simulink model "Simulation_P2_r2023a"  (R2023a)
settings: Solver=FixedStepAuto  StartTime=0.0  StopTime=10  FixedStep=1e-3  RelTol=1e-3  EnableMultiTasking=on
undefined symbols (not defined in the file): A0, A1, D0, D1, D10, D11, D12, D13, D2, D3, D4, D5, D6, D7, D8, D9, magnitude, PTA0, PTA1, PTA2, PTB2, PTB23, PTB3, PTB9, PTC16, PTC17, PTC2, PTC3, PTC4, PTD0, PTD1, PTD2, PTD3
libraries: frdmk64flib x20, etargetslib x18, dspstat3 x1
settings Model: ExtModeTrigDuration=5  Creator=sherr  LastModifiedBy=salihahussain
settings OptimizationCC: EnhancedBackFolding=on  PassReuseOutputArgsAs=Individual arguments  ZeroExternalMemoryAtStartup=off  ZeroInternalMemoryAtStartup=off  MaxStackSize=64  OptimizeBlockOrder=speed  DifferentSizesBufferReuse=on  OptimizationCustomize=off  EfficientTunableParamExpr=on
settings DebuggingCC: ParameterTunabilityLossMsg=error
settings HardwareCC: ProdBitPerPointer=32  ProdBitPerSizeT=32  ProdBitPerPtrDiffT=32  ProdLargestAtomicInteger=Long  ProdLargestAtomicFloat=Double  ProdWordSize=32  ProdHWDeviceType=ARM Compatible->ARM Cortex
settings SFSimCC: MATLABDynamicMemAlloc=off
settings RTWCC: Description=Embedded Coder  SystemTargetFile=ert.tlc  HardwareBoard=NXP FRDM-K64F  TLCOptions="-aInlineSetEventsForThisBaseRateFcn=TLC_FALSE -aSuppressMultiTaskScheduler=TLC_FALSE  -aRateBasedStepFcn=0"  TemplateMakefile=ert_default_tmf  Toolchain=GNU Tools for ARM Embedded Processors
settings CodeAppCC: ForceParamTrailComments=on  IgnoreCustomStorageClasses=off  OperatorAnnotations=on  SimulinkDataObjDesc=on  SFDataObjDesc=on  InsertBlockDesc=on
settings ERTTargetCC: ExtModeTransport=4  ExtModeMexFile=sendToCommService

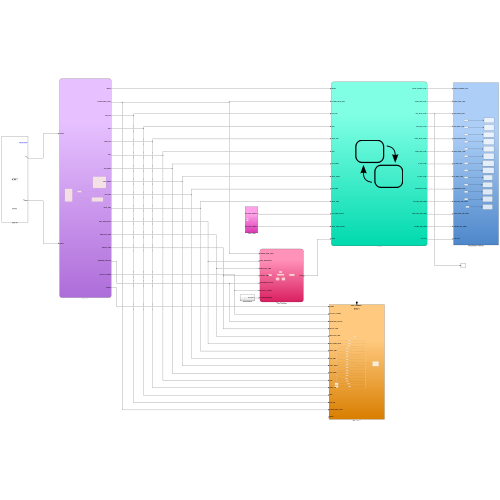
[thumbnail: Simulink's stored preview of the top-level diagram]
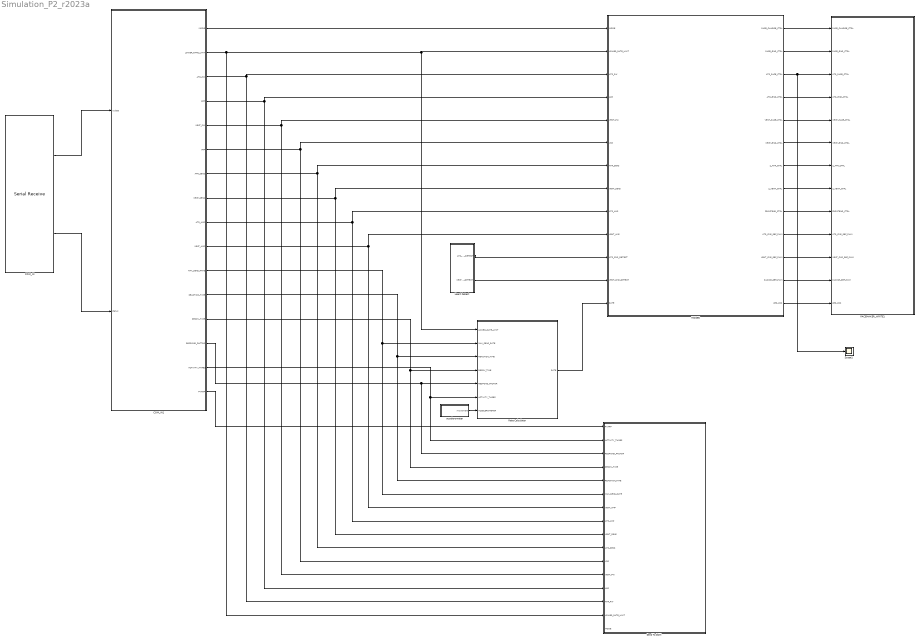
== system Simulation_P2_r2023a ==
  COM_IN : frdmk64flib/Serial Receive  SCIModule=0  Baudrate=uint32(9600)  Parity=None  StopBits=1  HardwareFlowControl=None  ByteOrder=LittleEndian  DataType=uint8  DataLength=10  BlockingMode=off  OutputStatus=on  SampleTime=0.1
  COM_IN1 : Stateflow chart  TreatAsAtomicUnit=on
      settings: PortSchema="{\"entries\":[{\"content\":{\"sides\":[{\"content\":{\"connectorIds\":[\"In1\",\"In2\"]},\"type\":\"ConnectorPlacement.EquallySpacedRectSide\",\"uuid\":\"bacdf752-87eb-4404-babc-2d3eecd8d2c0\"},{\"content\":{\"connectorIds\":[\"Out12\",\"Out7\",\"Out1\",\"Out2\",\"Out3\",\"Out4\",\"Out5\",\"Out6\",\"Out8\",\"Out9\",\"Out11\",\"Out13\",\"Out14\",\"Out15\",\"Out16\",\"Out10\"],\"side\":\"RIGHT\"},\"type\":\"ConnectorPlacement.EquallySpacedRectSide\",\"uuid\":\"87a5995d-41f9-45bd-b026-59ec7d01c35a\"},{\"content\":{\"side\":\"TOP\"},\"type\":\"ConnectorPlacement.EquallySpacedRectSide\",\"uuid\":\"9c1d1ff9-71c1-4ac7-ac77-ae13538ca481\"}]},\"type\":\"ConnectorPlacement.EquallySpacedConnector\",\"uuid\":\"f58684e7-fbf2-4992-a059-d31a56d65e02\"}],\"packageUris\":[\"http://schema.mathworks.com/mf0/Connector/R2020b\"],\"version\":\"1.0\"}"
  Heart Detect : Subsystem
  MODES : Stateflow chart  TreatAsAtomicUnit=on
  PACEMAKER_WRITE1 : Subsystem
  Rate Calculator : Stateflow chart  TreatAsAtomicUnit=on
      settings: PortSchema="{\"entries\":[{\"content\":{\"sides\":[{\"content\":{\"connectorIds\":[\"In3\",\"In7\",\"In5\",\"In4\",\"In1\",\"In2\",\"In6\"]},\"type\":\"ConnectorPlacement.EquallySpacedRectSide\",\"uuid\":\"c5d5357b-99af-427e-a4c2-6249b97164da\"},{\"content\":{\"connectorIds\":[\"Out1\"],\"side\":\"RIGHT\"},\"type\":\"ConnectorPlacement.EquallySpacedRectSide\",\"uuid\":\"358f3739-9c7f-4556-a3f3-e36ee066d1ea\"},{\"content\":{\"connectorIds\":[],\"side\":\"TOP\"},\"type\":\"ConnectorPlacement.EquallySpacedRectSide\",\"uuid\":\"e7873f65-b91d-40fa-bd89-8dce436ca138\"}]},\"type\":\"ConnectorPlacement.EquallySpacedConnector\",\"uuid\":\"f1b9a7e0-0d96-4ba5-9c87-c58b64bb2144\"}],\"packageUris\":[\"http://schema.mathworks.com/mf0/Connector/R2020b\"],\"version\":\"1.0\"}"
  Scope1 : Scope
  Send To DCM : Subsystem
  accelerometer : Subsystem
  wires:
  COM_IN/2 -> COM_IN1/2(status)
  COM_IN/1 -> COM_IN1/1(rxdata)
  MODES/10(ATR_CMP_REF_PWM) -> PACEMAKER_WRITE1/10(ATR_CMP_REF_PWM)
  MODES/2(PACE_GND_CTRL) -> PACEMAKER_WRITE1/2(PACE_GND_CTRL)
  MODES/6(VENT_GND_CTRL) -> PACEMAKER_WRITE1/6(VENT_GND_CTRL)
  MODES/11(VENT_CMP_REF_PWM) -> PACEMAKER_WRITE1/11(VENT_CMP_REF_PWM)
  MODES/9(FRONTEND_CTRL) -> PACEMAKER_WRITE1/9(FRONTEND_CTRL)
  MODES/13(LED_C22) -> PACEMAKER_WRITE1/13(LED_C22)
  MODES/1(PACE_CHARGE_CTRL) -> PACEMAKER_WRITE1/1(PACE_CHARGE_CTRL)
  MODES/7(Z_ATR_CTRL) -> PACEMAKER_WRITE1/7(Z_ATR_CTRL)
  MODES/4(ATR_GND_CTRL) -> PACEMAKER_WRITE1/4(ATR_GND_CTRL)
  MODES/5(VENT_PACE_CTRL) -> PACEMAKER_WRITE1/5(VENT_PACE_CTRL)
  MODES/12(PACING_REF_PWM) -> PACEMAKER_WRITE1/12(PACING_REF_PWM)
  MODES/8(Z_VENT_CTRL) -> PACEMAKER_WRITE1/8(Z_VENT_CTRL)
  MODES/3(ATR_PACE_CTRL) -> Scope1/1, PACEMAKER_WRITE1/3(ATR_PACE_CTRL)
  COM_IN1/9(VENT_AMP) -> Send To DCM/7(VENT_AMP), MODES/10(VENT_AMP)
  Heart Detect/1(ATR_CMP_DETECT) -> MODES/11(ATR_CMP_DETECT)
  Heart Detect/2(VENT_CMP_DETECT) -> MODES/12(VENT_CMP_DETECT)
  COM_IN1/12(MODE) -> MODES/1(MODE)
  COM_IN1/8(ATR_AMP) -> Send To DCM/8(ATR_AMP), MODES/9(ATR_AMP)
  COM_IN1/6(VENT_SENS) -> Send To DCM/9(VENT_SENS), MODES/8(VENT_SENS)
  COM_IN1/5(ATR_SENS) -> Send To DCM/10(ATR_SENS), MODES/7(ATR_SENS)
  COM_IN1/4(VRP) -> Send To DCM/11(VRP), MODES/6(VRP)
  COM_IN1/3(VENT_PW) -> Send To DCM/12(VENT_PW), MODES/5(VENT_PW)
  COM_IN1/2(ARP) -> Send To DCM/13(ARP), MODES/4(ARP)
  COM_IN1/1(ATR_PW) -> Send To DCM/14(ATR_PW), MODES/3(ATR_PW)
  COM_IN1/7(LOWER_RATE_LIMIT) -> Send To DCM/15(LOWER_RATE_LIMIT), Rate Calculator/3(LOWER_RATE_LIMIT), MODES/2(LOWER_RATE_LIMIT)
  COM_IN1/11(MAX_SENS_RATE) -> Send To DCM/6(MAX_SENS_RATE), Rate Calculator/7(MAX_SENS_RATE)
  COM_IN1/13(REACTION_TIME) -> Send To DCM/5(REACTION_TIME), Rate Calculator/5(REACTION_TIME)
  COM_IN1/14(RECOV_TIME) -> Send To DCM/4(RECOV_TIME), Rate Calculator/4(RECOV_TIME)
  COM_IN1/15(RESPOND_FACTOR) -> Send To DCM/3(RESPOND_FACTOR), Rate Calculator/1(RESPOND_FACTOR)
  COM_IN1/16(ACTIVITY_THRES) -> Send To DCM/2(ACTIVITY_THRES), Rate Calculator/2(ACTIVITY_THRES)
  accelerometer/1(movement) -> Rate Calculator/6(ACCELEROMETER)
  COM_IN1/10(PVARP) -> Send To DCM/1(PVARP)
  Rate Calculator/1(RATE) -> MODES/13(RATE)

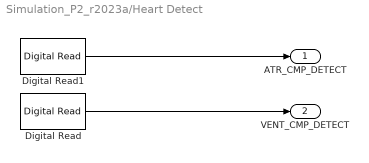
== system Simulation_P2_r2023a/Heart Detect ==
  Digital Read : frdmk64flib/Digital Read  Whichpin=PTC17 (D1)  SampleTime=-1
  Digital Read1 : frdmk64flib/Digital Read  Whichpin=PTC16 (D0)  SampleTime=-1
  ATR_CMP_DETECT : Outport
  VENT_CMP_DETECT : Outport  Port=2
  wires:
  Digital Read/1 -> VENT_CMP_DETECT/1
  Digital Read1/1 -> ATR_CMP_DETECT/1

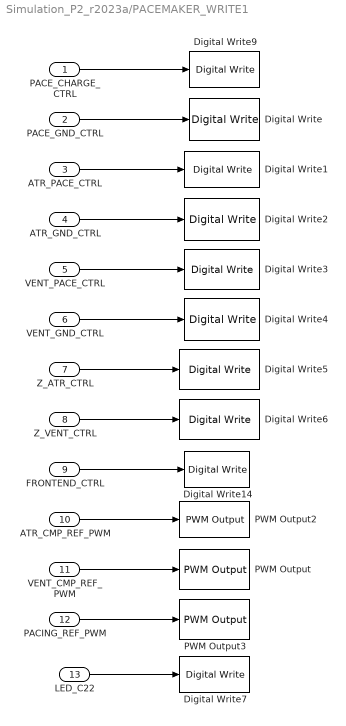
== system Simulation_P2_r2023a/PACEMAKER_WRITE1 ==
  PACE_CHARGE_CTRL : Inport
  PACE_GND_CTRL : Inport  Port=2
  ATR_PACE_CTRL : Inport  Port=3
  ATR_GND_CTRL : Inport  Port=4
  VENT_PACE_CTRL : Inport  Port=5
  VENT_GND_CTRL : Inport  Port=6
  Z_ATR_CTRL : Inport  Port=7
  Z_VENT_CTRL : Inport  Port=8
  FRONTEND_CTRL : Inport  Port=9
  ATR_CMP_REF_PWM : Inport  Port=10
  VENT_CMP_REF_PWM : Inport  Port=11
  PACING_REF_PWM : Inport  Port=12
  LED_C22 : Inport  Port=13
  Digital Write : frdmk64flib/Digital Write  Whichpin=PTD0 (D10)
  Digital Write1 : frdmk64flib/Digital Write  Whichpin=PTA0 (D8)
  Digital Write14 : frdmk64flib/Digital Write  Whichpin=PTD1 (D13)
  Digital Write2 : frdmk64flib/Digital Write  Whichpin=PTD2 (D11)
  Digital Write3 : frdmk64flib/Digital Write  Whichpin=PTC4 (D9)
  Digital Write4 : frdmk64flib/Digital Write  Whichpin=PTD3 (D12)
  Digital Write5 : frdmk64flib/Digital Write  Whichpin=PTB23 (D4)
  Digital Write6 : frdmk64flib/Digital Write  Whichpin=PTC3 (D7)
  Digital Write7 : frdmk64flib/Digital Write  Whichpin=BLUE_LED
  Digital Write9 : frdmk64flib/Digital Write  Whichpin=PTB9 (D2)
  PWM Output : frdmk64flib/PWM Output  Whichpin=PTA1 (D3)  InitialFrequency=2000  InitialDutyCycle=100
  PWM Output2 : frdmk64flib/PWM Output  Whichpin=PTC2 (D6)  InitialFrequency=2000  InitialDutyCycle=100
  PWM Output3 : frdmk64flib/PWM Output  Whichpin=PTA2 (D5)  InitialFrequency=2000  InitialDutyCycle=100
  wires:
  PACE_GND_CTRL/1 -> Digital Write/1
  ATR_CMP_REF_PWM/1 -> PWM Output2/1
  Z_ATR_CTRL/1 -> Digital Write5/1
  ATR_GND_CTRL/1 -> Digital Write2/1
  Z_VENT_CTRL/1 -> Digital Write6/1
  FRONTEND_CTRL/1 -> Digital Write14/1
  PACE_CHARGE_CTRL/1 -> Digital Write9/1
  VENT_GND_CTRL/1 -> Digital Write4/1
  PACING_REF_PWM/1 -> PWM Output3/1
  ATR_PACE_CTRL/1 -> Digital Write1/1
  VENT_CMP_REF_PWM/1 -> PWM Output/1
  VENT_PACE_CTRL/1 -> Digital Write3/1
  LED_C22/1 -> Digital Write7/1

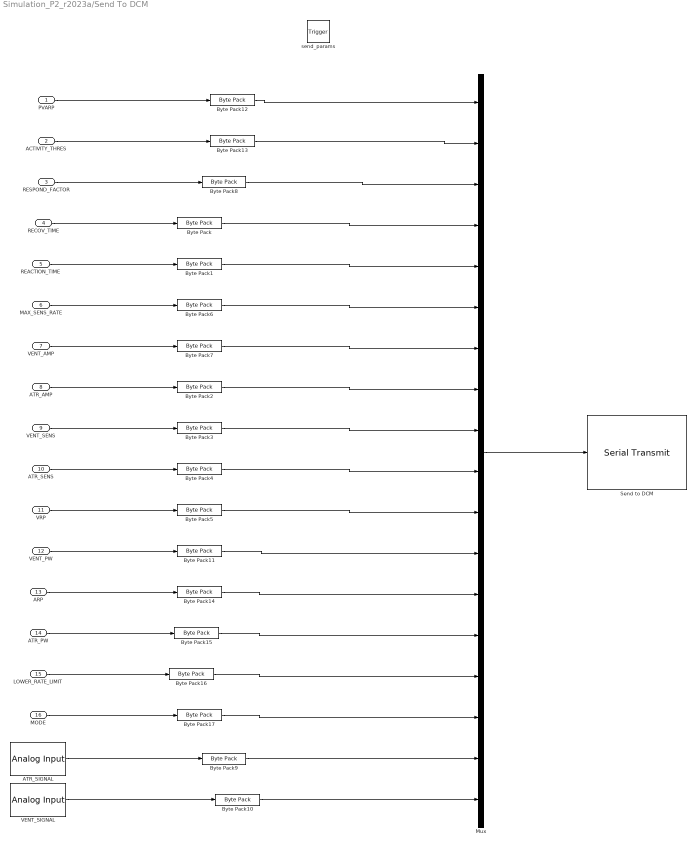
== system Simulation_P2_r2023a/Send To DCM ==
  PVARP : Inport
  ACTIVITY_THRES : Inport  Port=2
  RESPOND_FACTOR : Inport  Port=3
  RECOV_TIME : Inport  Port=4
  REACTION_TIME : Inport  Port=5
  MAX_SENS_RATE : Inport  Port=6
  VENT_AMP : Inport  Port=7
  ATR_AMP : Inport  Port=8
  VENT_SENS : Inport  Port=9
  ATR_SENS : Inport  Port=10
  VRP : Inport  Port=11
  VENT_PW : Inport  Port=12
  ARP : Inport  Port=13
  ATR_PW : Inport  Port=14
  LOWER_RATE_LIMIT : Inport  Port=15
  MODE : Inport  Port=16
  send_params : TriggerPort  TriggerType=function-call  IsSimulinkFunction=on  FunctionName=send_params  VariantControl=(inherit)  PortDimensions=1
  ATR_SIGNAL : frdmk64flib/Analog Input  Whichpin=PTB2 (A0)  SampleTime=-1
  Byte Pack{,1..3,6..7} (6 alike) : etargetslib/Byte Pack  datatypes={'single'}  byteAlign=1
  Byte Pack10 : etargetslib/Byte Pack  datatypes={'double'}  byteAlign=1
  Byte Pack{4..5,8,11..17} (10 alike) : etargetslib/Byte Pack  datatypes={'uint16'}  byteAlign=1
  Byte Pack9 : etargetslib/Byte Pack  datatypes={'double'}  byteAlign=1
  Mux : Mux  Inputs=18
  Send to DCM : frdmk64flib/Serial Transmit  SCIModule=0  Baudrate=uint32(9600)  Parity=None  StopBits=1  HardwareFlowControl=None  ByteOrder=LittleEndian  BlockingMode=on  OutputStatus=off
  VENT_SIGNAL : frdmk64flib/Analog Input  Whichpin=PTB3 (A1)  SampleTime=-1
  wires:
  PVARP/1 -> Byte Pack12/1
  ACTIVITY_THRES/1 -> Byte Pack13/1
  RECOV_TIME/1 -> Byte Pack/1
  Byte Pack/1 -> Mux/4
  REACTION_TIME/1 -> Byte Pack1/1
  Byte Pack1/1 -> Mux/5
  MAX_SENS_RATE/1 -> Byte Pack6/1
  VENT_AMP/1 -> Byte Pack7/1
  ATR_AMP/1 -> Byte Pack2/1
  Byte Pack2/1 -> Mux/8
  VENT_SENS/1 -> Byte Pack3/1
  Byte Pack3/1 -> Mux/9
  Byte Pack4/1 -> Mux/10
  ATR_SENS/1 -> Byte Pack4/1
  VRP/1 -> Byte Pack5/1
  Byte Pack5/1 -> Mux/11
  VENT_PW/1 -> Byte Pack11/1
  ARP/1 -> Byte Pack14/1
  ATR_PW/1 -> Byte Pack15/1
  LOWER_RATE_LIMIT/1 -> Byte Pack16/1
  MODE/1 -> Byte Pack17/1
  Mux/1 -> Send to DCM/1
  Byte Pack6/1 -> Mux/6
  Byte Pack7/1 -> Mux/7
  RESPOND_FACTOR/1 -> Byte Pack8/1
  ATR_SIGNAL/1 -> Byte Pack9/1
  VENT_SIGNAL/1 -> Byte Pack10/1
  Byte Pack10/1 -> Mux/18
  Byte Pack8/1 -> Mux/3
  Byte Pack9/1 -> Mux/17
  Byte Pack12/1 -> Mux/1
  Byte Pack13/1 -> Mux/2
  Byte Pack11/1 -> Mux/12
  Byte Pack14/1 -> Mux/13
  Byte Pack15/1 -> Mux/14
  Byte Pack16/1 -> Mux/15
  Byte Pack17/1 -> Mux/16

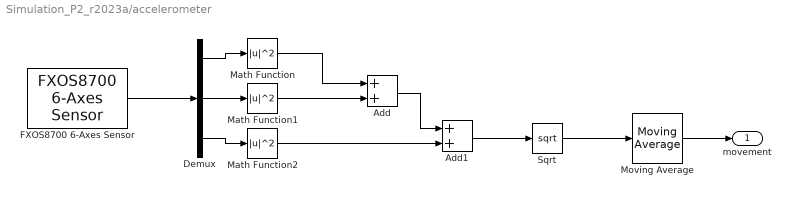
== system Simulation_P2_r2023a/accelerometer ==
  Add : Sum
  Add1 : Sum
  Demux : Demux  Outputs=3
  FXOS8700 6-Axes Sensor : frdmk64flib/FXOS8700 6-Axes Sensor  Activesensor=Accelerometer only  ODR=800Hz  HybridODR=400Hz  Accelfullrange=-4g to +4g  SampleTime=0.01
  Math Function : Math  Operator=magnitude^2
  Math Function1 : Math  Operator=magnitude^2
  Math Function2 : Math  Operator=magnitude^2
  Moving Average : dspstat3/Moving Average  Method=Sliding window  ForgettingFactorPort=off  SpecifyWindowLength=on  WindowLength=500  OverlapLength=499  AllowArbitraryInputLength=off  ForgettingFactor=0.9  SimulateUsing=Code generation
  Sqrt : Sqrt
  movement : Outport
  wires:
  Math Function/1 -> Add/1
  Math Function1/1 -> Add/2
  Math Function2/1 -> Add1/2
  Add/1 -> Add1/1
  Add1/1 -> Sqrt/1
  Sqrt/1 -> Moving Average/1
  Moving Average/1 -> movement/1
  FXOS8700 6-Axes Sensor/1 -> Demux/1
  Demux/1 -> Math Function/1
  Demux/2 -> Math Function1/1
  Demux/3 -> Math Function2/1

== stateflow chart Simulation_P2_r2023a/COM_IN1 ==
  note: Define datatype and size of each variables
  state SET_PARAM
    entry:
    MODE = typecast(rxdata(3:4),'uint16');
    LOWER_RATE_LIMIT = typecast(rxdata(5:6),'uint16');
    ATR_AMP = typecast(rxdata(7:10), 'single');
    ATR_PW = typecast(rxdata(11:14), 'single');
    VENT_AMP = typecast(rxdata(15:18), 'single');
    VENT_PW = typecast(rxdata(19:22), 'single');
    VRP = typecast(rxdata(23:24), 'uint16');
    ARP = typecast(rxdata(25:26), 'uint16');
    MAX_SENS_RATE = typecast(rxdata(27:28), 'uint16');
    ATR_SENS =typecast(rxdata(29:32), 'single');
    VENT_SENS = typecast(rxdata(33:36) ,'single');
    PVARP = typecast(rxdata(37:38), 'uint16');
    ACTIVITY_THRES = typecast(rxdata(39:40), 'uint16');
    REACTION_TIME = typecast(rxdata(41:42), 'uint16');
    RESPOND_FACTOR =typecast(rxdata(43:44), 'uint16');
    RECOV_TIME = typecast(rxdata(45:46), 'uint16');
  note: Set default values
  state INITIAL
    entry:
    MODE = 1; %select any mode
    LOWER_RATE_LIMIT = 60; %ppm
    ATR_AMP = 3.75;
    ATR_PW = 0.4;
    VENT_AMP = 3.75;
    VENT_PW = 0.4;
    VRP = 320;
    ARP = 250;
    MAX_SENS_RATE = 120;
    ATR_SENS = 0.075;%3.75
    VENT_SENS = 0.25;%3.75
    PVARP = 250;
    ACTIVITY_THRES = 0;
    REACTION_TIME = 30;
    RESPOND_FACTOR = 8;
    RECOV_TIME = 2;
  state STANDBY
    %waiting for COM
  state ECHO_PARAM
    entry:
    send_params();
  SET_PARAM -> STANDBY
  (default) -> INITIAL
  (junction 14) -> SET_PARAM [order 1] : [rxdata(2) == hex2dec('55')]
  INITIAL -> STANDBY
  STANDBY -> (junction 15) : [status == 0]
  (junction 15) -> (junction 14) : [rxdata(1) == hex2dec('16')]
  (junction 14) -> ECHO_PARAM [order 2] : [rxdata(2) == hex2dec('22')]
  ECHO_PARAM -> STANDBY
  data: rxdata input uint8; status input uint8; ATR_PW output uint16; ARP output uint16; VENT_PW output single; VRP output single; ATR_SENS output single; VENT_SENS output single; LOWER_RATE_LIMIT output uint16; ATR_AMP output single; VENT_AMP output single; PVARP output uint16; MAX_SENS_RATE output; MODE output uint16; REACTION_TIME output uint16; RECOV_TIME output uint16; RESPOND_FACTOR output uint16; ACTIVITY_THRES output uint16

== stateflow chart Simulation_P2_r2023a/MODES ==
  state INITIAL
    %Initial State
  state AOO [group]
    state CHARGING
      entry:
      %Begin Charging C22 Capacitor
      ATR_PACE_CTRL = 0
      VENT_PACE_CTRL = 0
      PACING_REF_PWM = 100*ATR_AMP/5
      PACE_CHARGE_CTRL = 1
      %Begin Discharging C21 Blocking Capacitor
      PACE_GND_CTRL = 1
      VENT_PACE_CTRL = 0
      Z_ATR_CTRL = 0
      Z_VENT_CTRL = 0
      ATR_PACE_CTRL = 0
      ATR_GND_CTRL = 1
      VENT_GND_CTRL = 0
      %Test
      LED_C22 = 1
    state DISCHARGING
      entry:
      %Discharge C22 into Atrium (AtrialPacing)
      %Begin Charging C21 Blocking Capacitor
      PACE_CHARGE_CTRL = 0
      PACE_GND_CTRL = 1
      ATR_PACE_CTRL = 1
      ATR_GND_CTRL = 0
      Z_ATR_CTRL = 0
      Z_VENT_CTRL = 0
      VENT_GND_CTRL = 0
      VENT_PACE_CTRL  = 0
    AOO.CHARGING -> AOO.DISCHARGING [order 1] : [after(((60000/LOWER_RATE_LIMIT)-ATR_PW), msec)]
    AOO.DISCHARGING -> AOO.CHARGING : [after(ATR_PW, msec)]
  state AAI [group]
    state PROXY
      entry:
      %Discharge C21 Blocking Capacitor
      PACE_GND_CTRL = true;
      VENT_PACE_CTRL = false;
      Z_ATR_CTRL = false;
      Z_VENT_CTRL = false;
      ATR_PACE_CTRL = false;
      ATR_GND_CTRL = true;
      VENT_GND_CTRL = false;
      %Charge C22
      ATR_PACE_CTRL = false;
      VENT_PACE_CTRL = false;
      PACING_REF_PWM = 100*ATR_AMP/5;
      PACE_CHARGE_CTRL = true;
    state CHARGING
      entry:
      %Sensing Circuitry
      FRONTEND_CTRL = HIGH
      %Assume appropriate PWM threshold
      ATR_CMP_REF_PWM = 100*ATR_AMP/5;
      VENT_CMP_REF_PWM = 0
      %Begin Charging C22 Capacitor
      ATR_PACE_CTRL = false;
      VENT_PACE_CTRL = false;
      PACING_REF_PWM = 100*ATR_AMP/5;
      PACE_CHARGE_CTRL = true;
      %Begin Discharging C21 Blocking Capacitor
      PACE_GND_CTRL = true;
      VENT_PACE_CTRL = false;
      Z_ATR_CTRL = false;
      Z_VENT_CTRL = false;
      ATR_PACE_CTRL = false;
      ATR_GND_CTRL = true;
      VENT_GND_CTRL = false;
    state DISCHARGING
      entry:
      %Discharge C22 into Atrium (Atrial Pacing)
      %Begin Charging Blocking Capacitor
      PACE_CHARGE_CTRL = LOW
      PACE_GND_CTRL = HIGH
      ATR_PACE_CTRL = HIGH
      ATR_GND_CTRL = LOW
      Z_ATR_CTRL = LOW
      Z_VENT_CTRL = LOW
      VENT_GND_CTRL = LOW
      VENT_PACE_CTRL  = LOW
    AAI.DISCHARGING -> AAI.PROXY : [after(ATR_PW, msec)]
    AAI.PROXY -> AAI.CHARGING : [after(ARP, msec)]
    (junction 116) -> AAI.PROXY : [after(LOWER_RATE_LIMIT, msec)]
    AAI.CHARGING -> (junction 116) [order 1] : [ATR_CMP_DETECT == HIGH]
    AAI.CHARGING -> AAI.DISCHARGING [order 2] : after(((60000/LOWER_RATE_LIMIT)-ATR_PW), msec)[ATR_CMP_DETECT == LOW]
  state VOO [group]
    state CHARGING
      entry:
      %Begin Charging C22 Capacitor
      ATR_PACE_CTRL = false;
      VENT_PACE_CTRL = false;
      PACING_REF_PWM = 100*VENT_AMP/5
      PACE_CHARGE_CTRL = true;
      %Begin Discharging C21 Blocking Capacitor
      PACE_GND_CTRL = true;
      VENT_PACE_CTRL = false;
      Z_ATR_CTRL = false;
      Z_VENT_CTRL = false;
      ATR_PACE_CTRL = false;
      ATR_GND_CTRL = false;
      VENT_GND_CTRL = true;
    state DISCHARGING
      entry:
      %Discharge C22 into Ventricle (Vent Pacing)
      %Begin Charging Blocking Capacitor
      PACE_CHARGE_CTRL = false;
      PACE_GND_CTRL = true;
      ATR_PACE_CTRL = false;
      ATR_GND_CTRL = false;
      Z_ATR_CTRL = false;
      Z_VENT_CTRL = false;
      VENT_GND_CTRL = false;
      VENT_PACE_CTRL  = true;
    VOO.CHARGING -> VOO.DISCHARGING [order 1] : [after(((60000/LOWER_RATE_LIMIT)-VENT_PW), msec)]
    VOO.DISCHARGING -> VOO.CHARGING : [after(VENT_PW, msec)]
  state VVI [group]
    state PROXY
      entry:
      %Step 1
      %Discharge C21 Blocking Capacitor
      PACE_GND_CTRL = HIGH
      VENT_PACE_CTRL = LOW
      Z_ATR_CTRL = LOW
      Z_VENT_CTRL = LOW
      ATR_PACE_CTRL = LOW
      ATR_GND_CTRL = LOW
      VENT_GND_CTRL = HIGH
      %Step 2
      %Charge C22
      ATR_PACE_CTRL = LOW
      VENT_PACE_CTRL = LOW
      PACING_REF_PWM = 100*VENT_AMP/5;
      PACE_CHARGE_CTRL = HIGH
    state CHARGING
      entry:
      %Sense Circuit
      FRONTEND_CTRL = true
      VENT_CMP_REF_PWM = (100*VENT_AMP)/5;
      ATR_CMP_REF_PWM = 0;
      %Begin Charging C22 Capacitor
      ATR_PACE_CTRL = LOW
      VENT_PACE_CTRL = LOW
      PACING_REF_PWM = 100*VENT_AMP/5;
      PACE_CHARGE_CTRL = HIGH
      %Begin Discharging Blocking Capacitor
      PACE_GND_CTRL = HIGH
      VENT_PACE_CTRL = LOW
      Z_ATR_CTRL = LOW
      Z_VENT_CTRL = LOW
      ATR_PACE_CTRL = LOW
      ATR_GND_CTRL = LOW
      VENT_GND_CTRL = HIGH
    state DISCHARGING
      entry:
      %Step 1:
      %Discharge C22 into Ventricle (Vent Pacing)
      %Begin Charging Blocking Capacitor
      PACE_CHARGE_CTRL = LOW
      PACE_GND_CTRL = HIGH
      ATR_PACE_CTRL = LOW
      ATR_GND_CTRL = LOW
      Z_ATR_CTRL = LOW
      Z_VENT_CTRL = LOW
      VENT_GND_CTRL = LOW
      VENT_PACE_CTRL  = HIGH
    VVI.DISCHARGING -> VVI.PROXY : [after(VENT_PW, msec)]
    VVI.PROXY -> VVI.CHARGING : [after(VRP, msec)]
    (junction 657) -> VVI.PROXY : [after(LOWER_RATE_LIMIT, msec)]
    VVI.CHARGING -> (junction 657) [order 1] : [VENT_CMP_DETECT ==  HIGH]
    VVI.CHARGING -> VVI.DISCHARGING [order 2] : after(((60000/LOWER_RATE_LIMIT)-VENT_PW), msec)[VENT_CMP_DETECT ==  LOW]
  state AOOR [group]
    state CHARGING
      entry:
      %Begin Charging C22 Capacitor
      ATR_PACE_CTRL = 0
      VENT_PACE_CTRL = 0
      PACING_REF_PWM = 100*ATR_AMP/5
      PACE_CHARGE_CTRL = 1
      %Begin Discharging C21 Blocking Capacitor
      PACE_GND_CTRL = 1
      VENT_PACE_CTRL = 0
      Z_ATR_CTRL = 0
      Z_VENT_CTRL = 0
      ATR_PACE_CTRL = 0
      ATR_GND_CTRL = 1
      VENT_GND_CTRL = 0
      %Test
      LED_C22 = 1
    state DISCHARGING
      entry:
      %Discharge C22 into Atrium (AtrialPacing)
      %Begin Charging C21 Blocking Capacitor
      PACE_CHARGE_CTRL = 0
      PACE_GND_CTRL = 1
      ATR_PACE_CTRL = 1
      ATR_GND_CTRL = 0
      Z_ATR_CTRL = 0
      Z_VENT_CTRL = 0
      VENT_GND_CTRL = 0
      VENT_PACE_CTRL  = 0
    AOOR.CHARGING -> AOOR.DISCHARGING [order 1] : [after(((60000/RATE)-ATR_PW), msec)]
    AOOR.DISCHARGING -> AOOR.CHARGING : [after(ATR_PW, msec)]
  state AAIR [group]
    state PROXY
      entry:
      %Discharge C21 Blocking Capacitor
      PACE_GND_CTRL = true;
      VENT_PACE_CTRL = false;
      Z_ATR_CTRL = false;
      Z_VENT_CTRL = false;
      ATR_PACE_CTRL = false;
      ATR_GND_CTRL = true;
      VENT_GND_CTRL = false;
      %Charge C22
      ATR_PACE_CTRL = false;
      VENT_PACE_CTRL = false;
      PACING_REF_PWM = 100*ATR_AMP/5;
      PACE_CHARGE_CTRL = true;
    state CHARGING
      entry:
      %Sensing Circuitry
      FRONTEND_CTRL = HIGH
      %Assume appropriate PWM threshold
      ATR_CMP_REF_PWM = 100*ATR_AMP/5;
      VENT_CMP_REF_PWM = 0
      %Begin Charging C22 Capacitor
      ATR_PACE_CTRL = false;
      VENT_PACE_CTRL = false;
      PACING_REF_PWM = 100*ATR_AMP/5;
      PACE_CHARGE_CTRL = true;
      %Begin Discharging C21 Blocking Capacitor
      PACE_GND_CTRL = true;
      VENT_PACE_CTRL = false;
      Z_ATR_CTRL = false;
      Z_VENT_CTRL = false;
      ATR_PACE_CTRL = false;
      ATR_GND_CTRL = true;
      VENT_GND_CTRL = false;
    state DISCHARGING
      entry:
      %Discharge C22 into Atrium (Atrial Pacing)
      %Begin Charging Blocking Capacitor
      PACE_CHARGE_CTRL = LOW
      PACE_GND_CTRL = HIGH
      ATR_PACE_CTRL = HIGH
      ATR_GND_CTRL = LOW
      Z_ATR_CTRL = LOW
      Z_VENT_CTRL = LOW
      VENT_GND_CTRL = LOW
      VENT_PACE_CTRL  = LOW
    AAIR.DISCHARGING -> AAIR.PROXY : [after(ATR_PW, msec)]
    AAIR.PROXY -> AAIR.CHARGING : [after(ARP, msec)]
    (junction 669) -> AAIR.PROXY : [after(RATE, msec)]
    AAIR.CHARGING -> (junction 669) [order 1] : [ATR_CMP_DETECT == HIGH]
    AAIR.CHARGING -> AAIR.DISCHARGING [order 2] : after(((60000/RATE)-ATR_PW), msec)[ATR_CMP_DETECT == LOW]
  state VOOR [group]
    state CHARGING
      entry:
      %Begin Charging C22 Capacitor
      ATR_PACE_CTRL = false;
      VENT_PACE_CTRL = false;
      PACING_REF_PWM = 100*VENT_AMP/5
      PACE_CHARGE_CTRL = true;
      %Begin Discharging C21 Blocking Capacitor
      PACE_GND_CTRL = true;
      VENT_PACE_CTRL = false;
      Z_ATR_CTRL = false;
      Z_VENT_CTRL = false;
      ATR_PACE_CTRL = false;
      ATR_GND_CTRL = false;
      VENT_GND_CTRL = true;
    state DISCHARGING
      entry:
      %Discharge C22 into Ventricle (Vent Pacing)
      %Begin Charging Blocking Capacitor
      PACE_CHARGE_CTRL = false;
      PACE_GND_CTRL = true;
      ATR_PACE_CTRL = false;
      ATR_GND_CTRL = false;
      Z_ATR_CTRL = false;
      Z_VENT_CTRL = false;
      VENT_GND_CTRL = false;
      VENT_PACE_CTRL  = true;
    VOOR.CHARGING -> VOOR.DISCHARGING [order 1] : [after(((60000/RATE)-VENT_PW), msec)]
    VOOR.DISCHARGING -> VOOR.CHARGING : [after(VENT_PW, msec)]
  state VVIR [group]
    state PROXY
      entry:
      %Step 1
      %Discharge C21 Blocking Capacitor
      PACE_GND_CTRL = HIGH
      VENT_PACE_CTRL = LOW
      Z_ATR_CTRL = LOW
      Z_VENT_CTRL = LOW
      ATR_PACE_CTRL = LOW
      ATR_GND_CTRL = LOW
      VENT_GND_CTRL = HIGH
      %Step 2
      %Charge C22
      ATR_PACE_CTRL = LOW
      VENT_PACE_CTRL = LOW
      PACING_REF_PWM = 100*VENT_AMP/5;
      PACE_CHARGE_CTRL = HIGH
    state CHARGING
      entry:
      %Sense Circuit
      FRONTEND_CTRL = true
      VENT_CMP_REF_PWM = (100*VENT_AMP)/5;
      ATR_CMP_REF_PWM = 0;
      %Begin Charging C22 Capacitor
      ATR_PACE_CTRL = LOW
      VENT_PACE_CTRL = LOW
      PACING_REF_PWM = 100*VENT_AMP/5;
      PACE_CHARGE_CTRL = HIGH
      %Begin Discharging Blocking Capacitor
      PACE_GND_CTRL = HIGH
      VENT_PACE_CTRL = LOW
      Z_ATR_CTRL = LOW
      Z_VENT_CTRL = LOW
      ATR_PACE_CTRL = LOW
      ATR_GND_CTRL = LOW
      VENT_GND_CTRL = HIGH
    state DISCHARGING
      entry:
      %Step 1:
      %Discharge C22 into Ventricle (Vent Pacing)
      %Begin Charging Blocking Capacitor
      PACE_CHARGE_CTRL = LOW
      PACE_GND_CTRL = HIGH
      ATR_PACE_CTRL = LOW
      ATR_GND_CTRL = LOW
      Z_ATR_CTRL = LOW
      Z_VENT_CTRL = LOW
      VENT_GND_CTRL = LOW
      VENT_PACE_CTRL  = HIGH
    VVIR.DISCHARGING -> VVIR.PROXY : [after(VENT_PW, msec)]
    VVIR.PROXY -> VVIR.CHARGING : [after(VRP, msec)]
    (junction 682) -> VVIR.PROXY : [after(RATE, msec)]
    VVIR.CHARGING -> (junction 682) [order 1] : [VENT_CMP_DETECT ==  HIGH]
    VVIR.CHARGING -> VVIR.DISCHARGING [order 2] : after(((60000/RATE)-VENT_PW), msec)[VENT_CMP_DETECT ==  LOW]
  INITIAL -> AOO.CHARGING [order 1] : [MODE == 1]
  INITIAL -> AAI.CHARGING [order 2] : [MODE == 2]
  INITIAL -> VOO.CHARGING [order 3] : [MODE == 3]
  INITIAL -> VVI.CHARGING [order 4] : [MODE == 4]
  INITIAL -> AOOR.CHARGING [order 5] : [MODE == 5]
  INITIAL -> AAIR.CHARGING [order 6] : [MODE == 6]
  INITIAL -> VOOR.CHARGING [order 7] : [MODE == 7]
  INITIAL -> VVIR.CHARGING [order 8] : [MODE == 8]
  VVIR.CHARGING -> INITIAL [order 3] : [MODE ~= 8]
  AOO.CHARGING -> INITIAL [order 2] : [MODE ~= 1]
  AOOR.CHARGING -> INITIAL [order 2] : [MODE ~= 5]
  AAI.CHARGING -> INITIAL [order 3] : [MODE ~= 2]
  VVI.CHARGING -> INITIAL [order 3] : [MODE ~= 4]
  AAIR.CHARGING -> INITIAL [order 3] : [MODE ~= 6]
  VOO.CHARGING -> INITIAL [order 2] : [MODE ~= 3]
  VOOR.CHARGING -> INITIAL [order 2] : [MODE ~= 7]
  (default) -> INITIAL
  data: PACE_CHARGE_CTRL output uint16; PACE_GND_CTRL output uint16; ATR_PACE_CTRL output uint16; ATR_GND_CTRL output uint16; VENT_PACE_CTRL output uint16; VENT_GND_CTRL output uint16; Z_ATR_CTRL output uint16; Z_VENT_CTRL output uint16; MODE input uint16; LOWER_RATE_LIMIT input uint16; ATR_PW input double; ARP input uint16; VENT_PW input double; VRP input uint16; HIGH local uint16 =1; LOW local uint16 =0; ATR_SENS input boolean; VENT_SENS input; ATR_AMP input; VENT_AMP input; ATR_CMP_DETECT input; FRONTEND_CTRL output; ATR_CMP_REF_PWM output; VENT_CMP_REF_PWM output; PACING_REF_PWM output; LED_C22 output; true local uint16 =1; false local uint16 =0; VENT_CMP_DETECT input; RATE input

== stateflow chart Simulation_P2_r2023a/Rate Calculator ==
  note: The initial rate is LRL
  state Begin
    entry:
    RATE = LOWER_RATE_LIMIT;
  note: THESE ARE THEIR COMMENTS
  note: Set step size. For example, if increase, how much should be increased.
  note: When the movement is below threshold, we set target to LRL.
  state Data_Check
    entry:
    reduce_step_size = (MAX_SENS_RATE-LOWER_RATE_LIMIT)/RECOV_TIME;
    increase_step_size = (MAX_SENS_RATE-LOWER_RATE_LIMIT)/REACTION_TIME;
  state Addition
    entry:
    target_rate = LOWER_RATE_LIMIT+RESPOND_FACTOR* (ACCELEROMETER-ACTIVITY_THRES);
    if(target_rate>=MAX_SENS_RATE)
    target_rate = MAX_SENS_RATE;
    end
  state Reduce
    entry:
    target_rate = LOWER_RATE_LIMIT;
  note: If movement larger than threshold, target rate calculated. Cannot exit MSR.
  note: If the current rate is less than the target rate, we add a step increse to it.
      | If the current rate is the same as target rate, no changes.
      | If the current rate is larger than the target rate, we subtract a step decrease.
  note: Checking every 0.1s
  state Change1
    entry:
    if(RATE< target_rate)
    RATE = RATE+ increase_step_size;
    elseif(RATE == target_rate)
    RATE = target_rate;
    elseif(RATE > target_rate)
    RATE = RATE - reduce_step_size;
    end
  state Change2
    entry:
    if(RATE< target_rate)
    RATE = RATE+ increase_step_size;
    elseif(RATE == target_rate)
    RATE = target_rate;
    elseif(RATE > target_rate)
    RATE = RATE - reduce_step_size;
    end
  note: If the current rate is less than the target rate, we add a step increse to it.
      | If the current rate is the same as target rate, no changes.
      | If the current rate is larger than the target rate, we subtract a step decrease.
  (default) -> Begin
  Begin -> Data_Check
  Data_Check -> Addition [order 1] : [ACCELEROMETER>=ACTIVITY_THRES]
  Addition -> Data_Check [order 2] : [ACCELEROMETER<ACTIVITY_THRES]
  Data_Check -> Reduce [order 2] : [ACCELEROMETER<ACTIVITY_THRES]
  Reduce -> Data_Check [order 1] : [ACCELEROMETER>=ACTIVITY_THRES]
  Change1 -> Reduce : [after(100,msec)]
  Reduce -> Change1 [order 2] : [after(100,msec)]
  Change2 -> Addition : [after(100,msec)]
  Addition -> Change2 [order 1] : [after(100,msec)]
  data: RESPOND_FACTOR input; ACTIVITY_THRES input; LOWER_RATE_LIMIT input; RATE output; RECOV_TIME input; REACTION_TIME input; ACCELEROMETER input; MAX_SENS_RATE input; increase_step_size local; target_rate local; reduce_step_size local
